simulink model "ADCS_LogicalArchitecture"  (R2024b)
settings: Solver=VariableStepAuto  StartTime=0.0  StopTime=10.0  RelTol=1e-3
settings Model: Creator=Ameya  LastModifiedBy=Ameya

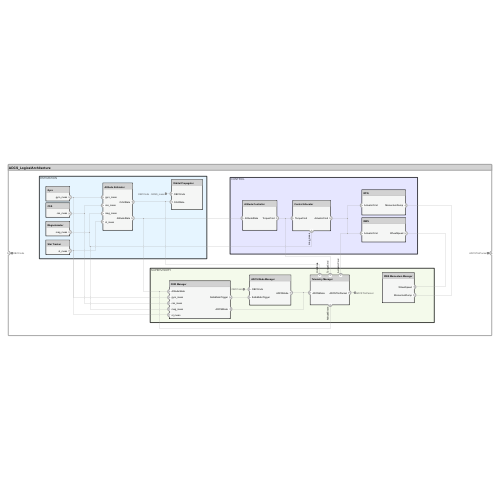
[thumbnail: Simulink's stored preview of the top-level diagram]
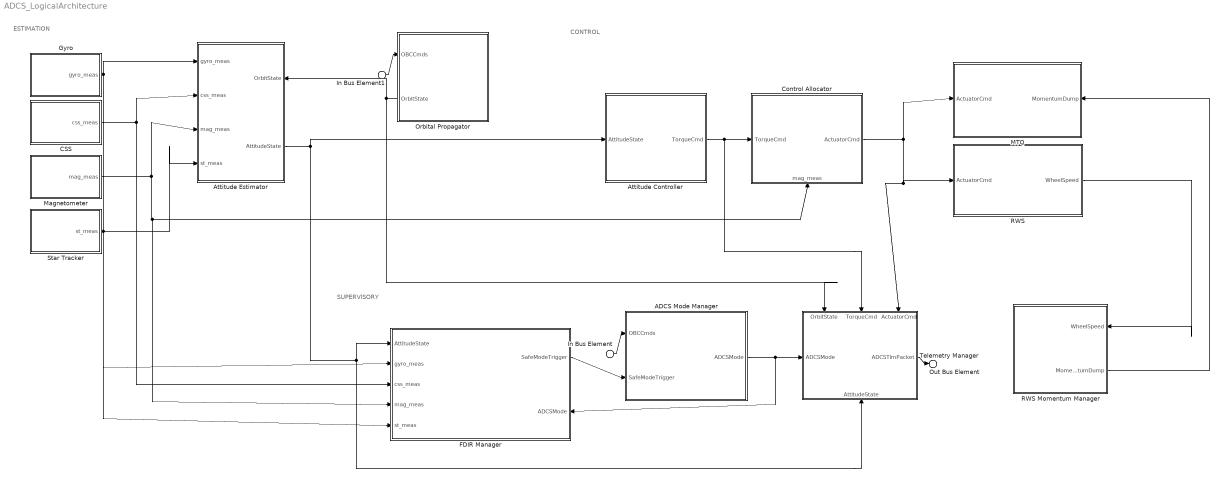
== system ADCS_LogicalArchitecture ==
  note: SUPERVISORY
  note: CONTROL
  note: ESTIMATION
  In Bus Element : Inport  PortName=OBCCmds
  In Bus Element1 : Inport  PortName=OBCCmds  Element=GNSS_meas
  ADCS Mode Manager : Subsystem
      settings: PortSchema="{\"entries\":[{\"content\":{\"headerSize\":26,\"margin\":15,\"minimumSpacing\":25,\"sides\":[{\"content\":{\"connectorIds\":[\"In1\",\"In2\"]},\"type\":\"ConnectorPlacement.EquallySpacedRectSide\",\"uuid\":\"f9f0631b-ecc8-46b5-bc4b-a7110d617b31\"},{\"content\":{\"connectorIds\":[\"Out1\"],\"side\":\"RIGHT\"},\"type\":\"ConnectorPlacement.EquallySpacedRectSide\",\"uuid\":\"e25df8eb-9b9e-42fa-ad3a-7152061d4b64\"},{\"content\":{\"side\":\"TOP\"},\"type\":\"ConnectorPlacement.EquallySpacedRectSide\",\"uuid\":\"cf5f9ecc-bb1a-43e9-8f34-af7d7746aec9\"}]},\"type\":\"ConnectorPlacement.EquallySpacedConnector\",\"uuid\":\"cfe5eff4-6c86-4801-a4da-a0246b82223c\"}],\"packageUris\":[\"http://schema.mathworks.com/mf0/Connector/R2020b\"],\"version\":\"1.0\"}"
  Attitude Controller : Subsystem
      settings: PortSchema="{\"entries\":[{\"content\":{\"headerSize\":26,\"margin\":15,\"minimumSpacing\":25,\"sides\":[{\"content\":{\"connectorIds\":[\"In1\"]},\"type\":\"ConnectorPlacement.EquallySpacedRectSide\",\"uuid\":\"f9f0631b-ecc8-46b5-bc4b-a7110d617b31\"},{\"content\":{\"connectorIds\":[\"Out1\"],\"side\":\"RIGHT\"},\"type\":\"ConnectorPlacement.EquallySpacedRectSide\",\"uuid\":\"e25df8eb-9b9e-42fa-ad3a-7152061d4b64\"},{\"content\":{\"side\":\"TOP\"},\"type\":\"ConnectorPlacement.EquallySpacedRectSide\",\"uuid\":\"cf5f9ecc-bb1a-43e9-8f34-af7d7746aec9\"}]},\"type\":\"ConnectorPlacement.EquallySpacedConnector\",\"uuid\":\"cfe5eff4-6c86-4801-a4da-a0246b82223c\"}],\"packageUris\":[\"http://schema.mathworks.com/mf0/Connector/R2020b\"],\"version\":\"1.0\"}"
  Attitude Estimator : Subsystem
      settings: PortSchema="{\"entries\":[{\"content\":{\"headerSize\":26,\"margin\":15,\"minimumSpacing\":25,\"sides\":[{\"content\":{\"connectorIds\":[\"In1\",\"In2\",\"In3\",\"In4\"]},\"type\":\"ConnectorPlacement.EquallySpacedRectSide\",\"uuid\":\"f9f0631b-ecc8-46b5-bc4b-a7110d617b31\"},{\"content\":{\"connectorIds\":[\"In5\",\"Out1\"],\"side\":\"RIGHT\"},\"type\":\"ConnectorPlacement.EquallySpacedRectSide\",\"uuid\":\"e25df8eb-9b9e-42fa-ad3a-7152061d4b64\"},{\"content\":{\"side\":\"TOP\"},\"type\":\"ConnectorPlacement.EquallySpacedRectSide\",\"uuid\":\"cf5f9ecc-bb1a-43e9-8f34-af7d7746aec9\"}]},\"type\":\"ConnectorPlacement.EquallySpacedConnector\",\"uuid\":\"cfe5eff4-6c86-4801-a4da-a0246b82223c\"}],\"packageUris\":[\"http://schema.mathworks.com/mf0/Connector/R2020b\"],\"version\":\"1.0\"}"
  CSS : Subsystem
      settings: PortSchema="{\"entries\":[{\"content\":{\"headerSize\":26,\"margin\":15,\"minimumSpacing\":25,\"sides\":[{\"content\":{},\"type\":\"ConnectorPlacement.EquallySpacedRectSide\",\"uuid\":\"f9f0631b-ecc8-46b5-bc4b-a7110d617b31\"},{\"content\":{\"connectorIds\":[\"Out1\"],\"side\":\"RIGHT\"},\"type\":\"ConnectorPlacement.EquallySpacedRectSide\",\"uuid\":\"e25df8eb-9b9e-42fa-ad3a-7152061d4b64\"},{\"content\":{\"side\":\"TOP\"},\"type\":\"ConnectorPlacement.EquallySpacedRectSide\",\"uuid\":\"cf5f9ecc-bb1a-43e9-8f34-af7d7746aec9\"}]},\"type\":\"ConnectorPlacement.EquallySpacedConnector\",\"uuid\":\"cfe5eff4-6c86-4801-a4da-a0246b82223c\"}],\"packageUris\":[\"http://schema.mathworks.com/mf0/Connector/R2020b\"],\"version\":\"1.0\"}"
  Control Allocator : Subsystem
      settings: PortSchema="{\"entries\":[{\"content\":{\"headerSize\":26,\"margin\":15,\"minimumSpacing\":25,\"sides\":[{\"content\":{\"connectorIds\":[\"In2\"]},\"type\":\"ConnectorPlacement.EquallySpacedRectSide\",\"uuid\":\"f9f0631b-ecc8-46b5-bc4b-a7110d617b31\"},{\"content\":{\"connectorIds\":[\"Out1\"],\"side\":\"RIGHT\"},\"type\":\"ConnectorPlacement.EquallySpacedRectSide\",\"uuid\":\"e25df8eb-9b9e-42fa-ad3a-7152061d4b64\"},{\"content\":{\"side\":\"TOP\"},\"type\":\"ConnectorPlacement.EquallySpacedRectSide\",\"uuid\":\"cf5f9ecc-bb1a-43e9-8f34-af7d7746aec9\"},{\"content\":{\"connectorIds\":[\"In1\"],\"side\":\"BOTTOM\"},\"type\":\"ConnectorPlacement.EquallySpacedRectSide\",\"uuid\":\"d7be6367-6943-46c2-9c06-66c0bf95472e\"}]},\"type\":\"ConnectorPlacement.EquallySpacedConnector\",\"uuid\":\"cfe5eff4-6c86-4801-a4da-a0246b82223c\"}],\"packageUris\":[\"http://schema.mathworks.com/mf0/Connector/R2020b\"],\"version\":\"1.0\"}"
  FDIR Manager : Subsystem
      settings: PortSchema="{\"entries\":[{\"content\":{\"headerSize\":26,\"margin\":15,\"minimumSpacing\":25,\"sides\":[{\"content\":{\"connectorIds\":[\"In6\",\"In2\",\"In3\",\"In4\",\"In5\"]},\"type\":\"ConnectorPlacement.EquallySpacedRectSide\",\"uuid\":\"f9f0631b-ecc8-46b5-bc4b-a7110d617b31\"},{\"content\":{\"connectorIds\":[\"Out1\",\"In1\"],\"side\":\"RIGHT\"},\"type\":\"ConnectorPlacement.EquallySpacedRectSide\",\"uuid\":\"e25df8eb-9b9e-42fa-ad3a-7152061d4b64\"},{\"content\":{\"side\":\"TOP\"},\"type\":\"ConnectorPlacement.EquallySpacedRectSide\",\"uuid\":\"cf5f9ecc-bb1a-43e9-8f34-af7d7746aec9\"}]},\"type\":\"ConnectorPlacement.EquallySpacedConnector\",\"uuid\":\"cfe5eff4-6c86-4801-a4da-a0246b82223c\"}],\"packageUris\":[\"http://schema.mathworks.com/mf0/Connector/R2020b\"],\"version\":\"1.0\"}"
  Gyro : Subsystem
      settings: PortSchema="{\"entries\":[{\"content\":{\"headerSize\":26,\"margin\":15,\"minimumSpacing\":25,\"sides\":[{\"content\":{},\"type\":\"ConnectorPlacement.EquallySpacedRectSide\",\"uuid\":\"f9f0631b-ecc8-46b5-bc4b-a7110d617b31\"},{\"content\":{\"connectorIds\":[\"Out1\"],\"side\":\"RIGHT\"},\"type\":\"ConnectorPlacement.EquallySpacedRectSide\",\"uuid\":\"e25df8eb-9b9e-42fa-ad3a-7152061d4b64\"},{\"content\":{\"side\":\"TOP\"},\"type\":\"ConnectorPlacement.EquallySpacedRectSide\",\"uuid\":\"cf5f9ecc-bb1a-43e9-8f34-af7d7746aec9\"}]},\"type\":\"ConnectorPlacement.EquallySpacedConnector\",\"uuid\":\"cfe5eff4-6c86-4801-a4da-a0246b82223c\"}],\"packageUris\":[\"http://schema.mathworks.com/mf0/Connector/R2020b\"],\"version\":\"1.0\"}"
  MTQ : Subsystem
      settings: PortSchema="{\"entries\":[{\"content\":{\"headerSize\":26,\"margin\":15,\"minimumSpacing\":25,\"sides\":[{\"content\":{\"connectorIds\":[\"In2\"]},\"type\":\"ConnectorPlacement.EquallySpacedRectSide\",\"uuid\":\"f9f0631b-ecc8-46b5-bc4b-a7110d617b31\"},{\"content\":{\"connectorIds\":[\"In1\"],\"side\":\"RIGHT\"},\"type\":\"ConnectorPlacement.EquallySpacedRectSide\",\"uuid\":\"e25df8eb-9b9e-42fa-ad3a-7152061d4b64\"},{\"content\":{\"side\":\"TOP\"},\"type\":\"ConnectorPlacement.EquallySpacedRectSide\",\"uuid\":\"cf5f9ecc-bb1a-43e9-8f34-af7d7746aec9\"}]},\"type\":\"ConnectorPlacement.EquallySpacedConnector\",\"uuid\":\"cfe5eff4-6c86-4801-a4da-a0246b82223c\"}],\"packageUris\":[\"http://schema.mathworks.com/mf0/Connector/R2020b\"],\"version\":\"1.0\"}"
  Magnetometer : Subsystem
      settings: PortSchema="{\"entries\":[{\"content\":{\"headerSize\":26,\"margin\":15,\"minimumSpacing\":25,\"sides\":[{\"content\":{},\"type\":\"ConnectorPlacement.EquallySpacedRectSide\",\"uuid\":\"f9f0631b-ecc8-46b5-bc4b-a7110d617b31\"},{\"content\":{\"connectorIds\":[\"Out1\"],\"side\":\"RIGHT\"},\"type\":\"ConnectorPlacement.EquallySpacedRectSide\",\"uuid\":\"e25df8eb-9b9e-42fa-ad3a-7152061d4b64\"},{\"content\":{\"side\":\"TOP\"},\"type\":\"ConnectorPlacement.EquallySpacedRectSide\",\"uuid\":\"cf5f9ecc-bb1a-43e9-8f34-af7d7746aec9\"}]},\"type\":\"ConnectorPlacement.EquallySpacedConnector\",\"uuid\":\"cfe5eff4-6c86-4801-a4da-a0246b82223c\"}],\"packageUris\":[\"http://schema.mathworks.com/mf0/Connector/R2020b\"],\"version\":\"1.0\"}"
  Orbital Propagator : Subsystem
      settings: PortSchema="{\"entries\":[{\"content\":{\"headerSize\":26,\"margin\":15,\"minimumSpacing\":25,\"sides\":[{\"content\":{\"connectorIds\":[\"In1\",\"Out1\"]},\"type\":\"ConnectorPlacement.EquallySpacedRectSide\",\"uuid\":\"f9f0631b-ecc8-46b5-bc4b-a7110d617b31\"},{\"content\":{\"side\":\"RIGHT\"},\"type\":\"ConnectorPlacement.EquallySpacedRectSide\",\"uuid\":\"e25df8eb-9b9e-42fa-ad3a-7152061d4b64\"},{\"content\":{\"side\":\"TOP\"},\"type\":\"ConnectorPlacement.EquallySpacedRectSide\",\"uuid\":\"cf5f9ecc-bb1a-43e9-8f34-af7d7746aec9\"}]},\"type\":\"ConnectorPlacement.EquallySpacedConnector\",\"uuid\":\"cfe5eff4-6c86-4801-a4da-a0246b82223c\"}],\"packageUris\":[\"http://schema.mathworks.com/mf0/Connector/R2020b\"],\"version\":\"1.0\"}"
  RWS : Subsystem
      settings: PortSchema="{\"entries\":[{\"content\":{\"headerSize\":26,\"margin\":15,\"minimumSpacing\":25,\"sides\":[{\"content\":{\"connectorIds\":[\"In1\"]},\"type\":\"ConnectorPlacement.EquallySpacedRectSide\",\"uuid\":\"f9f0631b-ecc8-46b5-bc4b-a7110d617b31\"},{\"content\":{\"connectorIds\":[\"Out1\"],\"side\":\"RIGHT\"},\"type\":\"ConnectorPlacement.EquallySpacedRectSide\",\"uuid\":\"e25df8eb-9b9e-42fa-ad3a-7152061d4b64\"},{\"content\":{\"side\":\"TOP\"},\"type\":\"ConnectorPlacement.EquallySpacedRectSide\",\"uuid\":\"cf5f9ecc-bb1a-43e9-8f34-af7d7746aec9\"},{\"content\":{\"side\":\"BOTTOM\"},\"type\":\"ConnectorPlacement.EquallySpacedRectSide\",\"uuid\":\"94257aed-66fb-4fc7-ac56-ba4ba4e593b7\"}]},\"type\":\"ConnectorPlacement.EquallySpacedConnector\",\"uuid\":\"cfe5eff4-6c86-4801-a4da-a0246b82223c\"}],\"packageUris\":[\"http://schema.mathworks.com/mf0/Connector/R2020b\"],\"version\":\"1.0\"}"
  RWS Momentum Manager : Subsystem
      settings: PortSchema="{\"entries\":[{\"content\":{\"headerSize\":26,\"margin\":15,\"minimumSpacing\":25,\"sides\":[{\"content\":{},\"type\":\"ConnectorPlacement.EquallySpacedRectSide\",\"uuid\":\"f9f0631b-ecc8-46b5-bc4b-a7110d617b31\"},{\"content\":{\"connectorIds\":[\"In1\",\"Out1\"],\"side\":\"RIGHT\"},\"type\":\"ConnectorPlacement.EquallySpacedRectSide\",\"uuid\":\"e25df8eb-9b9e-42fa-ad3a-7152061d4b64\"},{\"content\":{\"side\":\"TOP\"},\"type\":\"ConnectorPlacement.EquallySpacedRectSide\",\"uuid\":\"cf5f9ecc-bb1a-43e9-8f34-af7d7746aec9\"}]},\"type\":\"ConnectorPlacement.EquallySpacedConnector\",\"uuid\":\"cfe5eff4-6c86-4801-a4da-a0246b82223c\"}],\"packageUris\":[\"http://schema.mathworks.com/mf0/Connector/R2020b\"],\"version\":\"1.0\"}"
  Star Tracker : Subsystem
      settings: PortSchema="{\"entries\":[{\"content\":{\"headerSize\":26,\"margin\":15,\"minimumSpacing\":25,\"sides\":[{\"content\":{},\"type\":\"ConnectorPlacement.EquallySpacedRectSide\",\"uuid\":\"f9f0631b-ecc8-46b5-bc4b-a7110d617b31\"},{\"content\":{\"connectorIds\":[\"Out1\"],\"side\":\"RIGHT\"},\"type\":\"ConnectorPlacement.EquallySpacedRectSide\",\"uuid\":\"e25df8eb-9b9e-42fa-ad3a-7152061d4b64\"},{\"content\":{\"side\":\"TOP\"},\"type\":\"ConnectorPlacement.EquallySpacedRectSide\",\"uuid\":\"cf5f9ecc-bb1a-43e9-8f34-af7d7746aec9\"}]},\"type\":\"ConnectorPlacement.EquallySpacedConnector\",\"uuid\":\"cfe5eff4-6c86-4801-a4da-a0246b82223c\"}],\"packageUris\":[\"http://schema.mathworks.com/mf0/Connector/R2020b\"],\"version\":\"1.0\"}"
  Telemetry Manager : Subsystem
      settings: PortSchema="{\"entries\":[{\"content\":{\"headerSize\":26,\"margin\":15,\"minimumSpacing\":25,\"sides\":[{\"content\":{\"connectorIds\":[\"In2\"]},\"type\":\"ConnectorPlacement.EquallySpacedRectSide\",\"uuid\":\"f9f0631b-ecc8-46b5-bc4b-a7110d617b31\"},{\"content\":{\"connectorIds\":[\"Out1\"],\"side\":\"RIGHT\"},\"type\":\"ConnectorPlacement.EquallySpacedRectSide\",\"uuid\":\"e25df8eb-9b9e-42fa-ad3a-7152061d4b64\"},{\"content\":{\"connectorIds\":[\"In1\",\"In4\",\"In5\"],\"side\":\"TOP\"},\"type\":\"ConnectorPlacement.EquallySpacedRectSide\",\"uuid\":\"cf5f9ecc-bb1a-43e9-8f34-af7d7746aec9\"},{\"content\":{\"connectorIds\":[\"In3\"],\"side\":\"BOTTOM\"},\"type\":\"ConnectorPlacement.EquallySpacedRectSide\",\"uuid\":\"f9a234cd-4325-4b75-9a67-236778d7e2ed\"}]},\"type\":\"ConnectorPlacement.EquallySpacedConnector\",\"uuid\":\"cfe5eff4-6c86-4801-a4da-a0246b82223c\"}],\"packageUris\":[\"http://schema.mathworks.com/mf0/Connector/R2020b\"],\"version\":\"1.0\"}"
  Out Bus Element : Outport  PortName=ADCSTlmPacket
  wires:
  Orbital Propagator/1(OrbitState) -> Attitude Estimator/5(OrbitState), Telemetry Manager/1(OrbitState)
  Attitude Controller/1(TorqueCmd) -> Telemetry Manager/4(TorqueCmd), Control Allocator/2(TorqueCmd)
  In Bus Element/1 -> ADCS Mode Manager/1(OBCCmds)
  ADCS Mode Manager/1(ADCSMode) -> FDIR Manager/1(ADCSMode), Telemetry Manager/2(ADCSMode)
  Telemetry Manager/1(ADCSTlmPacket) -> Out Bus Element/1
  In Bus Element1/1 -> Orbital Propagator/1(OBCCmds)
  Gyro/1(gyro_meas) -> Attitude Estimator/1(gyro_meas), FDIR Manager/2(gyro_meas)
  CSS/1(css_meas) -> Attitude Estimator/2(css_meas), FDIR Manager/3(css_meas)
  Magnetometer/1(mag_meas) -> FDIR Manager/4(mag_meas), Control Allocator/1(mag_meas), Attitude Estimator/3(mag_meas)
  Star Tracker/1(st_meas) -> Attitude Estimator/4(st_meas), FDIR Manager/5(st_meas)
  Attitude Estimator/1(AttitudeState) -> Attitude Controller/1(AttitudeState), Telemetry Manager/3(AttitudeState), FDIR Manager/6(AttitudeState)
  Control Allocator/1(ActuatorCmd) -> Telemetry Manager/5(ActuatorCmd), RWS/1(ActuatorCmd), MTQ/2(ActuatorCmd)
  RWS/1(WheelSpeed) -> RWS Momentum Manager/1(WheelSpeed)
  RWS Momentum Manager/1(MomentumDump) -> MTQ/1(MomentumDump)
  FDIR Manager/1(SafeModeTrigger) -> ADCS Mode Manager/2(SafeModeTrigger)

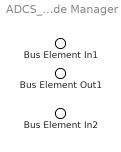
== system ADCS_LogicalArchitecture/ADCS Mode Manager ==
  Bus Element In1 : Inport  PortName=OBCCmds
  Bus Element In2 : Inport  Port=2  PortName=SafeModeTrigger
  Bus Element Out1 : Outport  PortName=ADCSMode

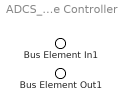
== system ADCS_LogicalArchitecture/Attitude Controller ==
  Bus Element In1 : Inport  PortName=AttitudeState
  Bus Element Out1 : Outport  PortName=TorqueCmd

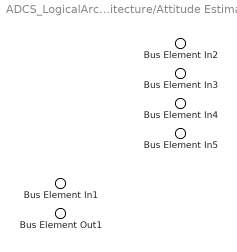
== system ADCS_LogicalArchitecture/Attitude Estimator ==
  Bus Element In2 : Inport  PortName=gyro_meas
  Bus Element In3 : Inport  Port=2  PortName=css_meas
  Bus Element In4 : Inport  Port=3  PortName=mag_meas
  Bus Element In5 : Inport  Port=4  PortName=st_meas
  Bus Element In1 : Inport  Port=5  PortName=OrbitState
  Bus Element Out1 : Outport  PortName=AttitudeState

== system ADCS_LogicalArchitecture/CSS ==
  Bus Element Out1 : Outport  PortName=css_meas

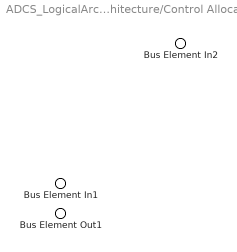
== system ADCS_LogicalArchitecture/Control Allocator ==
  Bus Element In2 : Inport  PortName=mag_meas
  Bus Element In1 : Inport  Port=2  PortName=TorqueCmd
  Bus Element Out1 : Outport  PortName=ActuatorCmd

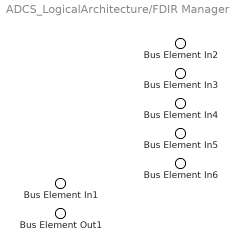
== system ADCS_LogicalArchitecture/FDIR Manager ==
  Bus Element In6 : Inport  PortName=ADCSMode
  Bus Element In2 : Inport  Port=2  PortName=gyro_meas
  Bus Element In3 : Inport  Port=3  PortName=css_meas
  Bus Element In4 : Inport  Port=4  PortName=mag_meas
  Bus Element In5 : Inport  Port=5  PortName=st_meas
  Bus Element In1 : Inport  Port=6  PortName=AttitudeState
  Bus Element Out1 : Outport  PortName=SafeModeTrigger

== system ADCS_LogicalArchitecture/Gyro ==
  Bus Element Out1 : Outport  PortName=gyro_meas

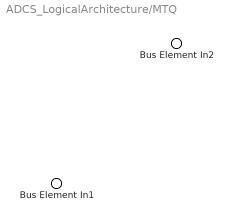
== system ADCS_LogicalArchitecture/MTQ ==
  Bus Element In2 : Inport  PortName=MomentumDump
  Bus Element In1 : Inport  Port=2  PortName=ActuatorCmd

== system ADCS_LogicalArchitecture/Magnetometer ==
  Bus Element Out1 : Outport  PortName=mag_meas

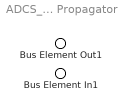
== system ADCS_LogicalArchitecture/Orbital Propagator ==
  Bus Element In1 : Inport  PortName=OBCCmds
  Bus Element Out1 : Outport  PortName=OrbitState

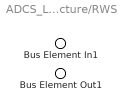
== system ADCS_LogicalArchitecture/RWS ==
  Bus Element In1 : Inport  PortName=ActuatorCmd
  Bus Element Out1 : Outport  PortName=WheelSpeed

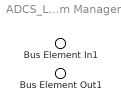
== system ADCS_LogicalArchitecture/RWS Momentum Manager ==
  Bus Element In1 : Inport  PortName=WheelSpeed
  Bus Element Out1 : Outport  PortName=MomentumDump

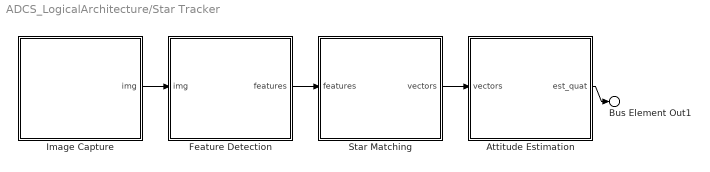
== system ADCS_LogicalArchitecture/Star Tracker ==
  Attitude Estimation : Subsystem
      settings: PortSchema="{\"entries\":[{\"content\":{\"headerSize\":26,\"margin\":15,\"minimumSpacing\":25,\"sides\":[{\"content\":{\"connectorIds\":[\"In1\"]},\"type\":\"ConnectorPlacement.EquallySpacedRectSide\",\"uuid\":\"f9f0631b-ecc8-46b5-bc4b-a7110d617b31\"},{\"content\":{\"connectorIds\":[\"Out1\"],\"side\":\"RIGHT\"},\"type\":\"ConnectorPlacement.EquallySpacedRectSide\",\"uuid\":\"e25df8eb-9b9e-42fa-ad3a-7152061d4b64\"},{\"content\":{\"side\":\"TOP\"},\"type\":\"ConnectorPlacement.EquallySpacedRectSide\",\"uuid\":\"cf5f9ecc-bb1a-43e9-8f34-af7d7746aec9\"}]},\"type\":\"ConnectorPlacement.EquallySpacedConnector\",\"uuid\":\"cfe5eff4-6c86-4801-a4da-a0246b82223c\"}],\"packageUris\":[\"http://schema.mathworks.com/mf0/Connector/R2020b\"],\"version\":\"1.0\"}"
  Feature Detection : Subsystem
      settings: PortSchema="{\"entries\":[{\"content\":{\"headerSize\":26,\"margin\":15,\"minimumSpacing\":25,\"sides\":[{\"content\":{\"connectorIds\":[\"In1\"]},\"type\":\"ConnectorPlacement.EquallySpacedRectSide\",\"uuid\":\"f9f0631b-ecc8-46b5-bc4b-a7110d617b31\"},{\"content\":{\"connectorIds\":[\"Out1\"],\"side\":\"RIGHT\"},\"type\":\"ConnectorPlacement.EquallySpacedRectSide\",\"uuid\":\"e25df8eb-9b9e-42fa-ad3a-7152061d4b64\"},{\"content\":{\"side\":\"TOP\"},\"type\":\"ConnectorPlacement.EquallySpacedRectSide\",\"uuid\":\"cf5f9ecc-bb1a-43e9-8f34-af7d7746aec9\"}]},\"type\":\"ConnectorPlacement.EquallySpacedConnector\",\"uuid\":\"cfe5eff4-6c86-4801-a4da-a0246b82223c\"}],\"packageUris\":[\"http://schema.mathworks.com/mf0/Connector/R2020b\"],\"version\":\"1.0\"}"
  Image Capture : Subsystem
      settings: PortSchema="{\"entries\":[{\"content\":{\"headerSize\":26,\"margin\":15,\"minimumSpacing\":25,\"sides\":[{\"content\":{},\"type\":\"ConnectorPlacement.EquallySpacedRectSide\",\"uuid\":\"f9f0631b-ecc8-46b5-bc4b-a7110d617b31\"},{\"content\":{\"connectorIds\":[\"Out1\"],\"side\":\"RIGHT\"},\"type\":\"ConnectorPlacement.EquallySpacedRectSide\",\"uuid\":\"e25df8eb-9b9e-42fa-ad3a-7152061d4b64\"},{\"content\":{\"side\":\"TOP\"},\"type\":\"ConnectorPlacement.EquallySpacedRectSide\",\"uuid\":\"cf5f9ecc-bb1a-43e9-8f34-af7d7746aec9\"}]},\"type\":\"ConnectorPlacement.EquallySpacedConnector\",\"uuid\":\"cfe5eff4-6c86-4801-a4da-a0246b82223c\"}],\"packageUris\":[\"http://schema.mathworks.com/mf0/Connector/R2020b\"],\"version\":\"1.0\"}"
  Star Matching : Subsystem
      settings: PortSchema="{\"entries\":[{\"content\":{\"headerSize\":26,\"margin\":15,\"minimumSpacing\":25,\"sides\":[{\"content\":{\"connectorIds\":[\"In1\"]},\"type\":\"ConnectorPlacement.EquallySpacedRectSide\",\"uuid\":\"f9f0631b-ecc8-46b5-bc4b-a7110d617b31\"},{\"content\":{\"connectorIds\":[\"Out1\"],\"side\":\"RIGHT\"},\"type\":\"ConnectorPlacement.EquallySpacedRectSide\",\"uuid\":\"e25df8eb-9b9e-42fa-ad3a-7152061d4b64\"},{\"content\":{\"side\":\"TOP\"},\"type\":\"ConnectorPlacement.EquallySpacedRectSide\",\"uuid\":\"cf5f9ecc-bb1a-43e9-8f34-af7d7746aec9\"}]},\"type\":\"ConnectorPlacement.EquallySpacedConnector\",\"uuid\":\"cfe5eff4-6c86-4801-a4da-a0246b82223c\"}],\"packageUris\":[\"http://schema.mathworks.com/mf0/Connector/R2020b\"],\"version\":\"1.0\"}"
  Bus Element Out1 : Outport  PortName=st_meas
  wires:
  Image Capture/1(img) -> Feature Detection/1(img)
  Feature Detection/1(features) -> Star Matching/1(features)
  Star Matching/1(vectors) -> Attitude Estimation/1(vectors)
  Attitude Estimation/1(est_quat) -> Bus Element Out1/1

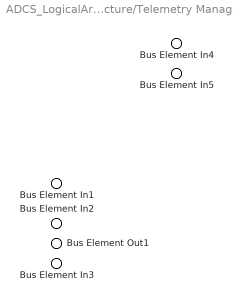
== system ADCS_LogicalArchitecture/Telemetry Manager ==
  Bus Element In5 : Inport  PortName=OrbitState
  Bus Element In4 : Inport  Port=2  PortName=ADCSMode
  Bus Element In1 : Inport  Port=3  PortName=AttitudeState
  Bus Element In2 : Inport  Port=4  PortName=TorqueCmd
  Bus Element In3 : Inport  Port=5  PortName=ActuatorCmd
  Bus Element Out1 : Outport  PortName=ADCSTlmPacket

== system ADCS_LogicalArchitecture/Star Tracker/Attitude Estimation ==
  Bus Element In1 : Inport  PortName=vectors
  Bus Element Out1 : Outport  PortName=est_quat

== system ADCS_LogicalArchitecture/Star Tracker/Feature Detection ==
  Bus Element In1 : Inport  PortName=img
  Bus Element Out1 : Outport  PortName=features

== system ADCS_LogicalArchitecture/Star Tracker/Image Capture ==
  Bus Element Out1 : Outport  PortName=img

== system ADCS_LogicalArchitecture/Star Tracker/Star Matching ==
  Bus Element In1 : Inport  PortName=features
  Bus Element Out1 : Outport  PortName=vectors
